simulink model "waypoint_control"  (Simulink 6.6)
settings: Solver=ode3  StartTime=0.0  StopTime=1000  FixedStep=T_step  RelTol=1e-3
values from neighbouring files (symbols this model uses):
  C_d_sea_surge = 200    [boat_constants.m]
  d_prop = .4572    (= 0.4572)    [boat_constants.m]
  K_t = 0.5    [boat_constants.m]
  lat_0 = 36.80611*pi/180    (= 0.642387804351)    [boat_constants.m]
  long_0 = -121.79639*pi/180    (= -2.12574802254)    [boat_constants.m]
  max_sea_state = 12    [boat_constants.m]
  phi_0 = 0    [boat_constants.m]
  proportional_band = .5    (= 0.5)    [boat_constants.m]
  rho_w = 1.03e3    (= 1030)    [boat_constants.m]
  roll_period = 3    [boat_constants.m]
  rudder_angle_dot_max = 10    [boat_constants.m]
  rudder_angle_max = 1    [boat_constants.m]
  sea_state = 0    [boat_constants.m]
  wheelbase = 3.27    [boat_constants.m]
undefined symbols (not defined in the file or in its folder): render_boat
libraries: simulink x4
settings Model: Creator=Administrator  LastModifiedBy=bmairs  SimulationMode=accelerator

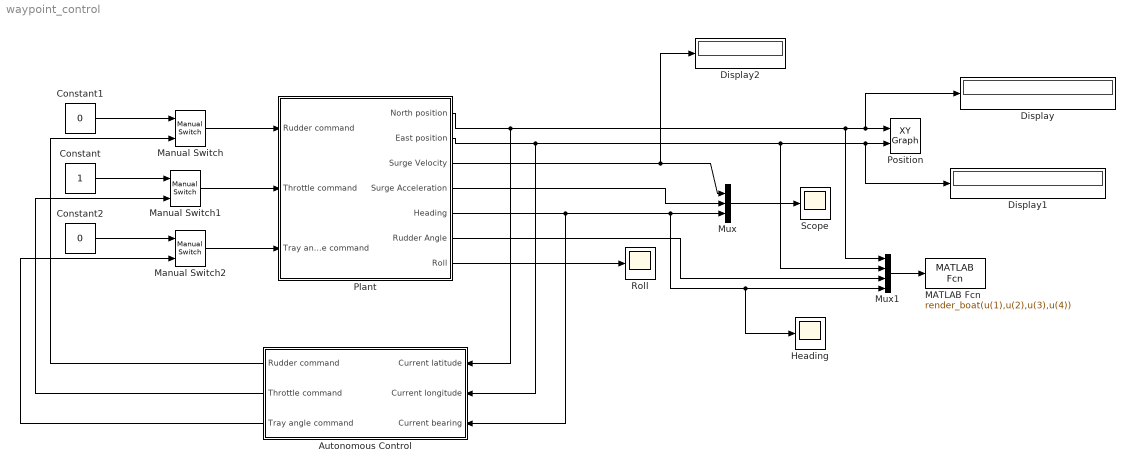
== system waypoint_control ==
  Autonomous Control : Subsystem  Orientation=left
  Constant : Constant
  Constant1 : Constant  Value=0
  Constant2 : Constant  Value=0
  Display : Display
  Display1 : Display
  Display2 : Display
  Heading : Scope
  MATLAB Fcn : MATLABFcn  MATLABFcn=render_boat(u(1),u(2),u(3),u(4))  OutputDimensions=0  Output1D=off
  Manual Switch : simulink/Signal Routing/Manual Switch  SystemSampleTime=-1  sw=0  action=0  varsize=off
  Manual Switch1 : simulink/Signal Routing/Manual Switch  SystemSampleTime=-1  sw=0  action=0  varsize=off
  Manual Switch2 : simulink/Signal Routing/Manual Switch  SystemSampleTime=-1  sw=0  action=0  varsize=off
  Mux : Mux  Inputs=3
  Mux1 : Mux
  Plant : Subsystem
  Position : simulink/Sinks/XY Graph  SystemSampleTime=-1  xmin=-200  xmax=200  ymin=-200  ymax=200  st=-1
  Roll : Scope
      settings: SaveName=ScopeData2
  Scope : Scope
      settings: YMin=-1.75  YMax=2
  wires:
  Plant/1(North position) -> Mux1/1, Position/1, Display/1, Autonomous Control/1(Current latitude)
  Plant/2(East position) -> Mux1/2, Position/2, Display1/1, Autonomous Control/2(Current longitude)
  Plant/3(Surge Velocity) -> Mux/1, Display2/1
  Plant/5(Heading) -> Mux1/4, Heading/1, Mux/3, Autonomous Control/3(Current bearing)
  Plant/4(Surge Acceleration) -> Mux/2
  Mux/1 -> Scope/1
  Mux1/1 -> MATLAB Fcn/1
  Plant/6(Rudder Angle) -> Mux1/3
  Plant/7(Roll) -> Roll/1
  Constant1/1 -> Manual Switch/1
  Manual Switch/1 -> Plant/1(Rudder command)
  Autonomous Control/1(Rudder command) -> Manual Switch/2
  Constant/1 -> Manual Switch1/1
  Manual Switch1/1 -> Plant/2(Throttle command)
  Autonomous Control/2(Throttle command) -> Manual Switch1/2
  Autonomous Control/3(Tray angle command) -> Manual Switch2/2
  Manual Switch2/1 -> Plant/3(Tray angle command)
  Constant2/1 -> Manual Switch2/1

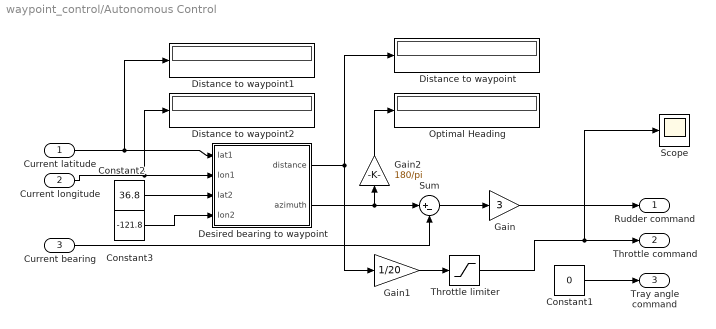
== system waypoint_control/Autonomous Control ==
  Current latitude : Inport
  Current longitude : Inport  Port=2
  Current bearing : Inport  Port=3
  Constant1 : Constant  Value=0
  Constant2 : Constant  Value=36.8
  Constant3 : Constant  Value=-121.8
  Desired bearing to waypoint : Stateflow chart
  Distance to waypoint : Display
  Distance to waypoint1 : Display
  Distance to waypoint2 : Display
  Gain : Gain  Gain=3
  Gain1 : Gain  Gain=1/20
  Gain2 : Gain  Orientation=up  Gain=180/pi
  Optimal Heading : Display
  Scope : Scope
      settings: SaveName=ScopeData3
  Sum : Sum  Inputs=|+-
  Throttle limiter : Saturate  UpperLimit=1  LowerLimit=0
  Rudder command : Outport
  Throttle command : Outport  Port=2
  Tray angle command : Outport  Port=3
  wires:
  Current latitude/1 -> Desired bearing to waypoint/1(lat1), Distance to waypoint1/1
  Current longitude/1 -> Desired bearing to waypoint/2(lon1), Distance to waypoint2/1
  Current bearing/1 -> Sum/2
  Throttle limiter/1 -> Throttle command/1, Scope/1
  Constant1/1 -> Tray angle command/1
  Sum/1 -> Gain/1
  Gain/1 -> Rudder command/1
  Desired bearing to waypoint/2(azimuth) -> Sum/1, Gain2/1
  Desired bearing to waypoint/1(distance) -> Distance to waypoint/1, Gain1/1
  Constant2/1 -> Desired bearing to waypoint/3(lat2)
  Constant3/1 -> Desired bearing to waypoint/4(lon2)
  Gain1/1 -> Throttle limiter/1
  Gain2/1 -> Optimal Heading/1

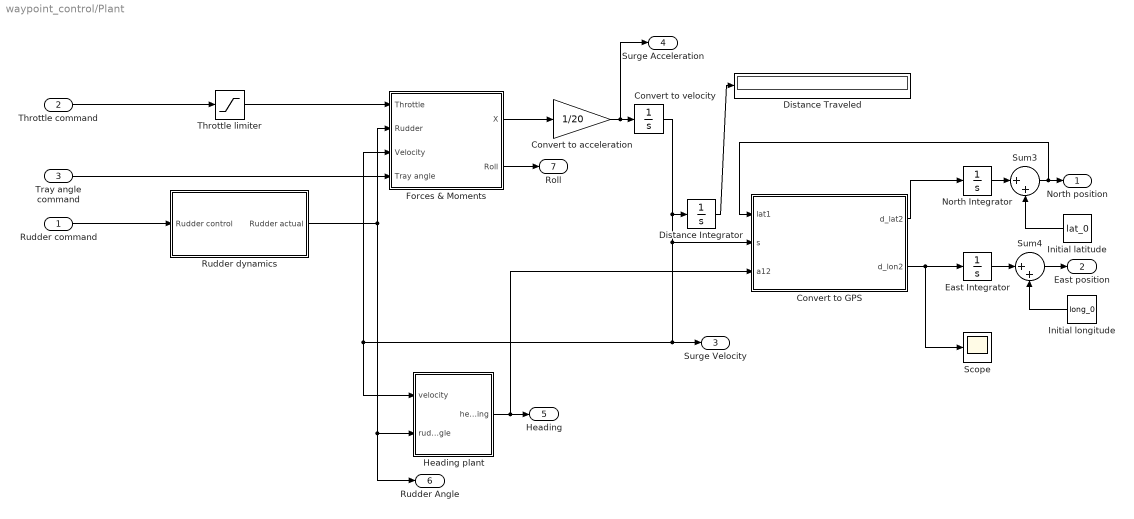
== system waypoint_control/Plant ==
  Rudder command : Inport
  Throttle command : Inport  Port=2
  Tray angle command : Inport  Port=3
  Convert to acceleration : Gain  Gain=1/20
  Convert to GPS : Stateflow chart
  Convert to velocity : Integrator
  Distance Integrator : Integrator
  Distance Traveled : Display
  East Integrator : Integrator
  Forces & Moments : Subsystem
  Heading plant : Subsystem
  Initial latitude : Constant  Orientation=left  Value=lat_0  SampleTime=-1
  Initial longitude : Constant  Orientation=left  Value=long_0  SampleTime=-1
  North Integrator : Integrator
  Rudder dynamics : Subsystem
  Scope : Scope
      settings: YMin=-1.75  YMax=2  SaveName=ScopeData4
  Sum3 : Sum  Inputs=|++
  Sum4 : Sum  Inputs=|++
  Throttle limiter : Saturate  UpperLimit=1  LowerLimit=0
  North position : Outport
  East position : Outport  Port=2
  Surge Velocity : Outport  Port=3
  Surge Acceleration : Outport  Port=4
  Heading : Outport  Port=5
  Rudder Angle : Outport  Port=6
  Roll : Outport  Port=7
  wires:
  Convert to velocity/1 -> Distance Integrator/1, Surge Velocity/1, Forces & Moments/3(Velocity), Heading plant/1(velocity), Convert to GPS/2(s)
  Forces & Moments/1(X) -> Convert to acceleration/1
  Throttle command/1 -> Throttle limiter/1
  Initial latitude/1 -> Sum3/2
  Sum3/1 -> North position/1, Convert to GPS/1(lat1)
  East Integrator/1 -> Sum4/1
  Sum4/1 -> East position/1
  Initial longitude/1 -> Sum4/2
  Throttle limiter/1 -> Forces & Moments/1(Throttle)
  Rudder command/1 -> Rudder dynamics/1(Rudder control)
  Rudder dynamics/1(Rudder actual) -> Forces & Moments/2(Rudder), Heading plant/2(rudder angle), Rudder Angle/1
  Forces & Moments/2(Roll) -> Roll/1
  Tray angle command/1 -> Forces & Moments/4(Tray angle)
  Distance Integrator/1 -> Distance Traveled/1
  Convert to acceleration/1 -> Surge Acceleration/1, Convert to velocity/1
  Heading plant/1(heading) -> Heading/1, Convert to GPS/3(a12)
  North Integrator/1 -> Sum3/1
  Convert to GPS/2(d_lon2) -> East Integrator/1, Scope/1
  Convert to GPS/1(d_lat2) -> North Integrator/1

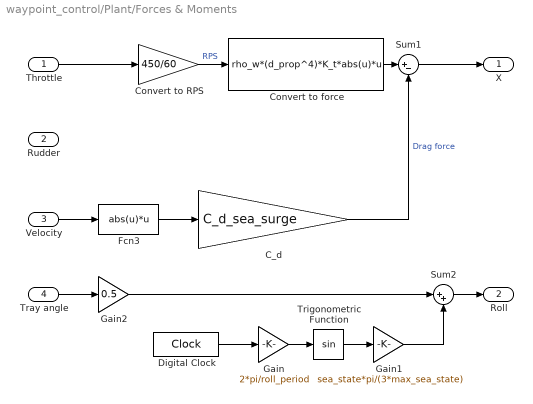
== system waypoint_control/Plant/Forces & Moments ==
  Throttle : Inport
  Rudder : Inport  Port=2
  Velocity : Inport  Port=3
  Tray angle : Inport  Port=4
  C_d : Gain  Gain=C_d_sea_surge
  Convert to RPS : Gain  Gain=450/60
  Convert to force : Fcn  Expr=rho_w*(d_prop^4)*K_t*abs(u)*u
  Digital Clock : DigitalClock  SampleTime=.01
  Fcn3 : Fcn  Expr=abs(u)*u
  Gain : Gain  Gain=2*pi/roll_period
  Gain1 : Gain  Gain=sea_state*pi/(3*max_sea_state)
  Gain2 : Gain  Gain=0.5
  Sum1 : Sum  Inputs=|+-
  Sum2 : Sum  Inputs=|++
  Trigonometric Function : Trigonometry
  X : Outport
  Roll : Outport  Port=2
  wires:
  Convert to RPS/1 -> Convert to force/1  "RPS"
  Fcn3/1 -> C_d/1
  C_d/1 -> Sum1/2  "Drag force"
  Convert to force/1 -> Sum1/1
  Velocity/1 -> Fcn3/1
  Throttle/1 -> Convert to RPS/1
  Sum1/1 -> X/1
  Digital Clock/1 -> Gain/1
  Gain/1 -> Trigonometric Function/1
  Trigonometric Function/1 -> Gain1/1
  Tray angle/1 -> Gain2/1
  Gain2/1 -> Sum2/1
  Gain1/1 -> Sum2/2
  Sum2/1 -> Roll/1

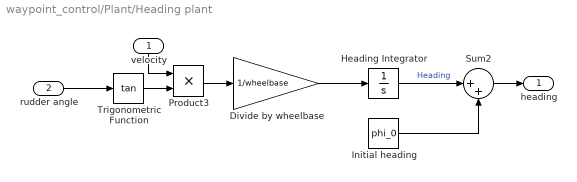
== system waypoint_control/Plant/Heading plant ==
  velocity : Inport  Orientation=down
  rudder angle : Inport  Port=2
  Divide by wheelbase : Gain  Gain=1/wheelbase
  Heading Integrator : Integrator
  Initial heading : Constant  Value=phi_0  SampleTime=-1
  Product3 : Product  RndMeth=Zero
  Sum2 : Sum  Inputs=|++
  Trigonometric Function : Trigonometry  Operator=tan  OutputSignalType=real
  heading : Outport
  wires:
  Trigonometric Function/1 -> Product3/2
  Product3/1 -> Divide by wheelbase/1
  Divide by wheelbase/1 -> Heading Integrator/1
  Heading Integrator/1 -> Sum2/1  "Heading"
  Initial heading/1 -> Sum2/2
  velocity/1 -> Product3/1
  rudder angle/1 -> Trigonometric Function/1
  Sum2/1 -> heading/1

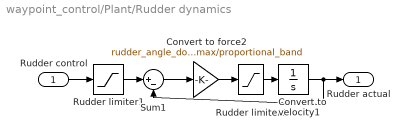
== system waypoint_control/Plant/Rudder dynamics ==
  Rudder control : Inport
  Convert to force2 : Gain  Gain=rudder_angle_dot_max/proportional_band
  Convert to velocity1 : Integrator  LimitOutput=on  UpperSaturationLimit=rudder_angle_max  LowerSaturationLimit=-rudder_angle_max
  Rudder limiter1 : Saturate  UpperLimit=rudder_angle_max  LowerLimit=-rudder_angle_max
  Rudder limiter2 : Saturate  UpperLimit=rudder_angle_dot_max  LowerLimit=-rudder_angle_dot_max
  Sum1 : Sum  Inputs=|+-
  Rudder actual : Outport
  wires:
  Convert to velocity1/1 -> Rudder actual/1, Sum1/2
  Sum1/1 -> Convert to force2/1
  Rudder limiter1/1 -> Sum1/1
  Rudder limiter2/1 -> Convert to velocity1/1
  Convert to force2/1 -> Rudder limiter2/1
  Rudder control/1 -> Rudder limiter1/1

== matlab function Autonomous Control/Desired bearing to waypoint ==
  data: lat1 input inherited; distance output inherited; lon1 input inherited; lat2 input inherited; lon2 input inherited; azimuth output inherited
%% - - - - - - - - - - - - - - - - - - - - - - - - - - - - - - - - - - - - - - - - - - - - - - - 
 %  Vincenty Inverse Solution of Geodesics on the Ellipsoid (c) Chris Veness 2002-2008           
 % - - - - - - - - - - - - - - - - - - - - - - - - - - - - - - - - - - - - - - - - - - - - - - - 
 %
 %
 % Calculate geodesic distance (in m) between two points specified by latitude/longitude 
 % (in numeric degrees) using Vincenty inverse formula for ellipsoids
%%
function [distance, azimuth] = distVincenty(lat1, lon1, lat2, lon2)
  a = 6378137;
  b = 6356752.3142;
  f = 1/298.257223563;  % WGS-84 ellipsiod
  L = (lon2-lon1)*pi/180;
  U1 = atan((1-f) * tan(lat1*pi/180));
  U2 = atan((1-f) * tan(lat2*pi/180));
  sinU1 = sin(U1);
  cosU1 = cos(U1);
  sinU2 = sin(U2);
  cosU2 = cos(U2);
  
  lambda = L;
  iterLimit = 100;
  while true;
    sinLambda = sin(lambda);
    cosLambda = cos(lambda);
    sinSigma = sqrt((cosU2*sinLambda) * (cosU2*sinLambda) + (cosU1*sinU2-sinU1*cosU2*cosLambda) * (cosU1*sinU2-sinU1*cosU2*cosLambda));
    if sinSigma==0; 
        distance = 0; % co-incident points
        azimuth = 0;
        return;
    end
    cosSigma = sinU1*sinU2 + cosU1*cosU2*cosLambda;
    sigma = atan2(sinSigma, cosSigma);
    sinAlpha = cosU1 * cosU2 * sinLambda / sinSigma;
    cosSqAlpha = 1 - sinAlpha*sinAlpha;
    cos2SigmaM = cosSigma - 2*sinU1*sinU2/cosSqAlpha;
    if isNaN(cos2SigmaM);
        cos2SigmaM = 0;  % equatorial line: cosSqAlpha=0 (§6)
    end
    C = f/16*cosSqAlpha*(4+f*(4-3*cosSqAlpha));
    lambdaP = lambda;
    lambda = L + (1-C) * f * sinAlpha * (sigma + C*sinSigma*(cos2SigmaM+C*cosSigma*(-1+2*cos2SigmaM*cos2SigmaM)));
    iterLimit = iterLimit - 1;
    if abs(lambda-lambdaP) > 1e-12 && iterLimit > 0;
        break;
    end
  end

  if iterLimit == 0;
      distance = NaN;  %formula failed to converge
      azimuth = NaN;
      return;
  end

  uSq = cosSqAlpha * (a*a - b*b) / (b*b);
  A = 1 + uSq/16384*(4096+uSq*(-768+uSq*(320-175*uSq)));
  B = uSq/1024 * (256+uSq*(-128+uSq*(74-47*uSq)));
  deltaSigma = B*sinSigma*(cos2SigmaM+B/4*(cosSigma*(-1+2*cos2SigmaM*cos2SigmaM) - B/6*cos2SigmaM*(-3+4*sinSigma*sinSigma)*(-3+4*cos2SigmaM*cos2SigmaM)));
  distance = b*A*(sigma-deltaSigma);
  
  % Calculate the heading that would be a direct course from point 1 to point 2
  azimuth = atan2(cosU2*sin(lambda), cosU1*sinU2 - sinU1*cosU2*cos(lambda));
 end

== matlab function Plant/Convert to GPS ==
  data: lat1 input inherited; d_lat2 output inherited; s input inherited; d_lon2 output inherited; a12 input inherited
function [d_lat2,d_lon2] = vreckon(lat1,s,a12)
% RECKON - Using the WGS-84 Earth ellipsoid, travel a given distance along
%          a given azimuth starting at a given initial point, and return
%          the endpoint within a few millimeters of accuracy, using
%          Vincenty's algorithm.
%
% USAGE:
% [lat2,lon2] = vreckon(lat1, lon1, s, a12)
%
% VARIABLES:
% lat1 = inital latitude (degrees)
% lon1 = initial longitude (degrees)
% s    = distance (meters)
% a12  = intial azimuth (degrees)
% lat2, lon2 = second point (degrees)
% a21  = reverse azimuth (degrees), at final point facing back toward the
%        intial point
%
% This algorithm was modified slightly for use with embedded Matlab and
% for the constraints of its use in this project by Bryant Mairs 07/2009
%
% Original algorithm source:
% T. Vincenty, "Direct and Inverse Solutions of Geodesics on the Ellipsoid
% with Application of Nested Equations", Survey Review, vol. 23, no. 176,
% April 1975, pp 88-93.
% Available at: http://www.ngs.noaa.gov/PUBS_LIB/inverse.pdf
%
% Notes: 
% (1) The Vincenty reckoning algorithm was transcribed verbatim into
%     JavaScript by Chris Veness. It was modified and translated to Matlab
%     by Michael Kleder. Mr. Veness's website is:
%     http://www.movable-type.co.uk/scripts/latlong-vincenty-direct.html
% (2) Error correcting code, polar error corrections, WGS84 ellipsoid
%     parameters, testing, and comments by Michael Kleder.
% (3) By convention, when starting at a pole, the longitude of the initial
%     point (otherwise meaningless) determines the longitude line along
%     which to traverse, and hence the longitude of the final point.
% (4) The convention noted in (3) above creates a discrepancy with VDIST
%     when the the intial or final point is at a pole. In the VDIST
%     function, when traversing from a pole, the azimuth is  0 when
%     heading away from the south pole and 180 when heading away from the
%     north pole. In contrast, this VRECKON function uses the azimuth as
%     noted in (3) above when traversing away form a pole.
% (5) In testing, where the traversal subtends no more than 178 degrees,
%     this function correctly inverts the VDIST function to within 0.2
%     millimeters of distance, 5e-10 degrees of forward azimuth,
%     and 5e-10 degrees of reverse azimuth. Precision reduces as test
%     points approach antipodal because the precision of VDIST is reduced
%     for nearly antipodal points. (A warning is given by VDIST.)
% (6) Tested but no warranty. Use at your own risk.
% (7) Ver 1.0, Michael Kleder, November 2007

a = 6378137; % semimajor axis
b = 6356752.31424518; % semiminor axis
f = 1/298.257223563; % flattening coefficient
lat1_orig = lat1;
lat1   = lat1 * .1745329251994329577e-1; % intial latitude in radians
% correct for errors at exact poles by adjusting 0.6 millimeters:
if abs(pi/2-abs(lat1)) < 1e-10;
    lat1 = sign(lat1)*(pi/2-(1e-10));
end
alpha1 = a12;% * .1745329251994329577e-1; % inital azimuth in radians
sinAlpha1 = sin(alpha1);
cosAlpha1 = cos(alpha1);
tanU1 = (1-f) * tan(lat1);
cosU1 = 1 / sqrt(1 + tanU1*tanU1);
sinU1 = tanU1*cosU1;
sigma1 = atan2(tanU1, cosAlpha1);
sinAlpha = cosU1 * sinAlpha1;
cosSqAlpha = 1 - sinAlpha*sinAlpha;
uSq = cosSqAlpha * (a*a - b*b) / (b*b);
A = 1 + uSq/16384*(4096+uSq*(-768+uSq*(320-175*uSq)));
B = uSq/1024 * (256+uSq*(-128+uSq*(74-47*uSq)));
sigma = s / (b*A);
sigmaP = 2*pi;
cos2SigmaM = cos(2*sigma1 + sigma);
sinSigma = sin(sigma);
cosSigma = cos(sigma);
while (abs(sigma-sigmaP) > 1e-18)
    cos2SigmaM = cos(2*sigma1 + sigma);
    sinSigma = sin(sigma);
    cosSigma = cos(sigma);
    deltaSigma = B*sinSigma*(cos2SigmaM+B/4*(cosSigma*(-1+...
        2*cos2SigmaM*cos2SigmaM)-...
        B/6*cos2SigmaM*(-3+4*sinSigma*sinSigma)*(-3+...
        4*cos2SigmaM*cos2SigmaM)));
    sigmaP = sigma;
    sigma = s / (b*A) + deltaSigma;
end
tmp = sinU1*sinSigma - cosU1*cosSigma*cosAlpha1;
lat2 = atan2(sinU1*cosSigma + cosU1*sinSigma*cosAlpha1,...
    (1-f)*sqrt(sinAlpha*sinAlpha + tmp*tmp));
lambda = atan2(sinSigma*sinAlpha1, cosU1*cosSigma - ...
    sinU1*sinSigma*cosAlpha1);
C = f/16*cosSqAlpha*(4+f*(4-3*cosSqAlpha));
L = lambda - (1-C) * f * sinAlpha * (sigma + C*sinSigma*(cos2SigmaM+...
    C*cosSigma*(-1+2*cos2SigmaM*cos2SigmaM)));
% output degrees
d_lat2 = lat2*57.295779513082322865 - lat1_orig;
d_lon2 = L*57.295779513082322865;
d_lon2 = mod(d_lon2,360); % follow [0,360] convention
return
